simulink model "loop_test"  (R2017b)
settings: Solver=FixedStepDiscrete  StartTime=0.0  StopTime=10.0  RelTol=1e-3  EnableMultiTasking=on
settings Model: Creator=Mitchell Cassaday  LastModifiedBy=Mitchell Cassaday

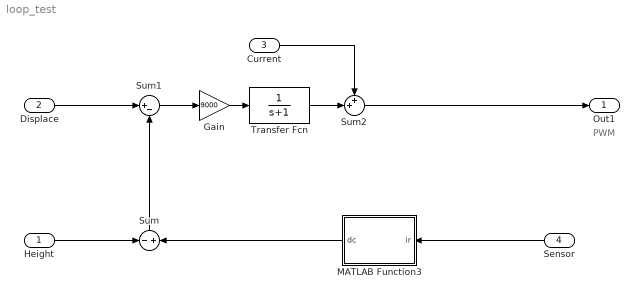
== system loop_test ==
  note: PWM
  Height : Inport
  Displace : Inport  Port=2
  Current : Inport  Port=3
  Sensor : Inport  Port=4
  Gain : Gain  Gain=9000
  MATLAB Function3 : MATLAB Function  TreatAsAtomicUnit=on
  Sum : Sum  Inputs=-|+
  Sum1 : Sum  Inputs=|+-
  Sum2 : Sum  Inputs=++|
  Transfer Fcn : TransferFcn  Denominator=[1 1]
  Out1 : Outport
  wires:
  MATLAB Function3/1(dc) -> Sum/2
  Height/1 -> Sum/1
  Sum/1 -> Sum1/2
  Sum1/1 -> Gain/1
  Displace/1 -> Sum1/1
  Current/1 -> Sum2/1
  Sum2/1 -> Out1/1
  Gain/1 -> Transfer Fcn/1
  Transfer Fcn/1 -> Sum2/2
  Sensor/1 -> MATLAB Function3/1(ir)

== matlab function loop_test/MATLAB Function3 ==
  data: ir input; dc output
function dc = fcn(ir)
    min_ir = cast(220,'single');
    max_ir = cast(3860,'single');
    dc = cast(((cast(ir,'single')-min_ir) ./ (max_ir-min_ir) .* 100.0),'int32');
